simulink model "ResearchPaper4Fig9"  (R2015b)
settings: Solver=VariableStepAuto  StartTime=0.0  StopTime=10.0  RelTol=1e-3
libraries: xbsIndex_r4 x942, commfilt2 x1, commrandsrc3 x1, commdigbbndam3 x1
(part 6 of 6)

== system ResearchPaper4Fig9/PseudoConv. RVTDNN6/Output Neuron1/Weight Update4 for O.N ==
  eta'grad : Inport
  o1 : Inport  Port=2
  AddSub : xbsIndex_r4/AddSub  mode=Addition  use_carryin=off  use_carryout=off  en=off  latency=0  precision=Full  arith_type=Unsigned  n_bits=16  bin_pt=14  quantization=Truncate  overflow=Wrap  use_behavioral_HDL=off  hw_selection=Fabric  pipelined=off  dbl_ovrd=off  block_type=addsub
  Mult : xbsIndex_r4/Mult  precision=Full  arith_type="Signed  (2's comp)"  n_bits=16  bin_pt=14  quantization=Truncate  overflow=Wrap  en=off  latency=0  use_behavioral_HDL=off  opt=Speed  use_embedded=on  optimum_pipeline=off  pipeline=on  dbl_ovrd=off  use_rpm=on  placement_style=Triangular  block_type=mult
  Register : xbsIndex_r4/Register  init=0  rst=off  en=off  dbl_ovrd=off  block_type=register
  w11 : Outport
  wires:
  Mult/1 -> AddSub/1
  Register/1 -> w11/1, AddSub/2
  AddSub/1 -> Register/1
  eta'grad/1 -> Mult/1
  o1/1 -> Mult/2

== system ResearchPaper4Fig9/PseudoConv. RVTDNN6/Output Neuron1/Weight Update5 for O.N ==
  eta'grad : Inport
  o1 : Inport  Port=2
  AddSub : xbsIndex_r4/AddSub  mode=Addition  use_carryin=off  use_carryout=off  en=off  latency=0  precision=Full  arith_type=Unsigned  n_bits=16  bin_pt=14  quantization=Truncate  overflow=Wrap  use_behavioral_HDL=off  hw_selection=Fabric  pipelined=off  dbl_ovrd=off  block_type=addsub
  Mult : xbsIndex_r4/Mult  precision=Full  arith_type="Signed  (2's comp)"  n_bits=16  bin_pt=14  quantization=Truncate  overflow=Wrap  en=off  latency=0  use_behavioral_HDL=off  opt=Speed  use_embedded=on  optimum_pipeline=off  pipeline=on  dbl_ovrd=off  use_rpm=on  placement_style=Triangular  block_type=mult
  Register : xbsIndex_r4/Register  init=0  rst=off  en=off  dbl_ovrd=off  block_type=register
  w11 : Outport
  wires:
  Mult/1 -> AddSub/1
  Register/1 -> w11/1, AddSub/2
  AddSub/1 -> Register/1
  eta'grad/1 -> Mult/1
  o1/1 -> Mult/2

== system ResearchPaper4Fig9/PseudoConv. RVTDNN6/Output Neuron1/Weight Update6 for O.N ==
  eta'grad : Inport
  o1 : Inport  Port=2
  AddSub : xbsIndex_r4/AddSub  mode=Addition  use_carryin=off  use_carryout=off  en=off  latency=0  precision=Full  arith_type=Unsigned  n_bits=16  bin_pt=14  quantization=Truncate  overflow=Wrap  use_behavioral_HDL=off  hw_selection=Fabric  pipelined=off  dbl_ovrd=off  block_type=addsub
  Mult : xbsIndex_r4/Mult  precision=Full  arith_type="Signed  (2's comp)"  n_bits=16  bin_pt=14  quantization=Truncate  overflow=Wrap  en=off  latency=0  use_behavioral_HDL=off  opt=Speed  use_embedded=on  optimum_pipeline=off  pipeline=on  dbl_ovrd=off  use_rpm=on  placement_style=Triangular  block_type=mult
  Register : xbsIndex_r4/Register  init=0  rst=off  en=off  dbl_ovrd=off  block_type=register
  w11 : Outport
  wires:
  Mult/1 -> AddSub/1
  Register/1 -> w11/1, AddSub/2
  AddSub/1 -> Register/1
  eta'grad/1 -> Mult/1
  o1/1 -> Mult/2

== system ResearchPaper4Fig9/PseudoConv. RVTDNN6/Output Neuron2/Bias Update for O.N ==
  grad : Inport
  AddSub : xbsIndex_r4/AddSub  mode=Addition  use_carryin=off  use_carryout=off  en=off  latency=0  precision=Full  arith_type=Unsigned  n_bits=16  bin_pt=14  quantization=Truncate  overflow=Wrap  use_behavioral_HDL=off  hw_selection=Fabric  pipelined=off  dbl_ovrd=off  block_type=addsub
  Register : xbsIndex_r4/Register  init=0  rst=off  en=off  dbl_ovrd=off  block_type=register
  w10 : Outport
  wires:
  Register/1 -> w10/1, AddSub/2
  AddSub/1 -> Register/1
  grad/1 -> AddSub/1

== system ResearchPaper4Fig9/PseudoConv. RVTDNN6/Output Neuron2/Sum ==
  In1 : Inport
  In2 : Inport  Port=2
  In3 : Inport  Port=3
  In4 : Inport  Port=4
  In5 : Inport  Port=5
  In6 : Inport  Port=6
  In7 : Inport  Port=7
  AddSub{,1..5} (6 alike) : xbsIndex_r4/AddSub  mode=Addition  use_carryin=off  use_carryout=off  en=off  latency=0  precision=Full  arith_type=Unsigned  n_bits=16  bin_pt=14  quantization=Truncate  overflow=Wrap  use_behavioral_HDL=off  hw_selection=Fabric  pipelined=off  dbl_ovrd=off  block_type=addsub
  Out : Outport
  wires:
  AddSub4/1 -> AddSub5/2
  AddSub3/1 -> AddSub5/1
  In7/1 -> AddSub4/2
  AddSub1/1 -> AddSub3/2
  AddSub2/1 -> AddSub4/1
  In1/1 -> AddSub/1
  In6/1 -> AddSub2/2
  In2/1 -> AddSub/2
  In4/1 -> AddSub1/2
  AddSub/1 -> AddSub3/1
  In5/1 -> AddSub2/1
  AddSub5/1 -> Out/1
  In3/1 -> AddSub1/1

== system ResearchPaper4Fig9/PseudoConv. RVTDNN6/Output Neuron2/Weight Update1 for O.N ==
  eta'grad : Inport
  o1 : Inport  Port=2
  AddSub : xbsIndex_r4/AddSub  mode=Addition  use_carryin=off  use_carryout=off  en=off  latency=0  precision=Full  arith_type=Unsigned  n_bits=16  bin_pt=14  quantization=Truncate  overflow=Wrap  use_behavioral_HDL=off  hw_selection=Fabric  pipelined=off  dbl_ovrd=off  block_type=addsub
  Mult : xbsIndex_r4/Mult  precision=Full  arith_type="Signed  (2's comp)"  n_bits=16  bin_pt=14  quantization=Truncate  overflow=Wrap  en=off  latency=0  use_behavioral_HDL=off  opt=Speed  use_embedded=on  optimum_pipeline=off  pipeline=on  dbl_ovrd=off  use_rpm=on  placement_style=Triangular  block_type=mult
  Register : xbsIndex_r4/Register  init=0  rst=off  en=off  dbl_ovrd=off  block_type=register
  w11 : Outport
  wires:
  Mult/1 -> AddSub/1
  Register/1 -> w11/1, AddSub/2
  AddSub/1 -> Register/1
  eta'grad/1 -> Mult/1
  o1/1 -> Mult/2

== system ResearchPaper4Fig9/PseudoConv. RVTDNN6/Output Neuron2/Weight Update2 for O.N ==
  eta'grad : Inport
  o1 : Inport  Port=2
  AddSub : xbsIndex_r4/AddSub  mode=Addition  use_carryin=off  use_carryout=off  en=off  latency=0  precision=Full  arith_type=Unsigned  n_bits=16  bin_pt=14  quantization=Truncate  overflow=Wrap  use_behavioral_HDL=off  hw_selection=Fabric  pipelined=off  dbl_ovrd=off  block_type=addsub
  Mult : xbsIndex_r4/Mult  precision=Full  arith_type="Signed  (2's comp)"  n_bits=16  bin_pt=14  quantization=Truncate  overflow=Wrap  en=off  latency=0  use_behavioral_HDL=off  opt=Speed  use_embedded=on  optimum_pipeline=off  pipeline=on  dbl_ovrd=off  use_rpm=on  placement_style=Triangular  block_type=mult
  Register : xbsIndex_r4/Register  init=0  rst=off  en=off  dbl_ovrd=off  block_type=register
  w11 : Outport
  wires:
  Mult/1 -> AddSub/1
  Register/1 -> w11/1, AddSub/2
  AddSub/1 -> Register/1
  eta'grad/1 -> Mult/1
  o1/1 -> Mult/2

== system ResearchPaper4Fig9/PseudoConv. RVTDNN6/Output Neuron2/Weight Update3 for O.N ==
  eta'grad : Inport
  o1 : Inport  Port=2
  AddSub : xbsIndex_r4/AddSub  mode=Addition  use_carryin=off  use_carryout=off  en=off  latency=0  precision=Full  arith_type=Unsigned  n_bits=16  bin_pt=14  quantization=Truncate  overflow=Wrap  use_behavioral_HDL=off  hw_selection=Fabric  pipelined=off  dbl_ovrd=off  block_type=addsub
  Mult : xbsIndex_r4/Mult  precision=Full  arith_type="Signed  (2's comp)"  n_bits=16  bin_pt=14  quantization=Truncate  overflow=Wrap  en=off  latency=0  use_behavioral_HDL=off  opt=Speed  use_embedded=on  optimum_pipeline=off  pipeline=on  dbl_ovrd=off  use_rpm=on  placement_style=Triangular  block_type=mult
  Register : xbsIndex_r4/Register  init=0  rst=off  en=off  dbl_ovrd=off  block_type=register
  w11 : Outport
  wires:
  Mult/1 -> AddSub/1
  Register/1 -> w11/1, AddSub/2
  AddSub/1 -> Register/1
  eta'grad/1 -> Mult/1
  o1/1 -> Mult/2

== system ResearchPaper4Fig9/PseudoConv. RVTDNN6/Output Neuron2/Weight Update4 for O.N ==
  eta'grad : Inport
  o1 : Inport  Port=2
  AddSub : xbsIndex_r4/AddSub  mode=Addition  use_carryin=off  use_carryout=off  en=off  latency=0  precision=Full  arith_type=Unsigned  n_bits=16  bin_pt=14  quantization=Truncate  overflow=Wrap  use_behavioral_HDL=off  hw_selection=Fabric  pipelined=off  dbl_ovrd=off  block_type=addsub
  Mult : xbsIndex_r4/Mult  precision=Full  arith_type="Signed  (2's comp)"  n_bits=16  bin_pt=14  quantization=Truncate  overflow=Wrap  en=off  latency=0  use_behavioral_HDL=off  opt=Speed  use_embedded=on  optimum_pipeline=off  pipeline=on  dbl_ovrd=off  use_rpm=on  placement_style=Triangular  block_type=mult
  Register : xbsIndex_r4/Register  init=0  rst=off  en=off  dbl_ovrd=off  block_type=register
  w11 : Outport
  wires:
  Mult/1 -> AddSub/1
  Register/1 -> w11/1, AddSub/2
  AddSub/1 -> Register/1
  eta'grad/1 -> Mult/1
  o1/1 -> Mult/2

== system ResearchPaper4Fig9/PseudoConv. RVTDNN6/Output Neuron2/Weight Update5 for O.N ==
  eta'grad : Inport
  o1 : Inport  Port=2
  AddSub : xbsIndex_r4/AddSub  mode=Addition  use_carryin=off  use_carryout=off  en=off  latency=0  precision=Full  arith_type=Unsigned  n_bits=16  bin_pt=14  quantization=Truncate  overflow=Wrap  use_behavioral_HDL=off  hw_selection=Fabric  pipelined=off  dbl_ovrd=off  block_type=addsub
  Mult : xbsIndex_r4/Mult  precision=Full  arith_type="Signed  (2's comp)"  n_bits=16  bin_pt=14  quantization=Truncate  overflow=Wrap  en=off  latency=0  use_behavioral_HDL=off  opt=Speed  use_embedded=on  optimum_pipeline=off  pipeline=on  dbl_ovrd=off  use_rpm=on  placement_style=Triangular  block_type=mult
  Register : xbsIndex_r4/Register  init=0  rst=off  en=off  dbl_ovrd=off  block_type=register
  w11 : Outport
  wires:
  Mult/1 -> AddSub/1
  Register/1 -> w11/1, AddSub/2
  AddSub/1 -> Register/1
  eta'grad/1 -> Mult/1
  o1/1 -> Mult/2

== system ResearchPaper4Fig9/PseudoConv. RVTDNN6/Output Neuron2/Weight Update6 for O.N ==
  eta'grad : Inport
  o1 : Inport  Port=2
  AddSub : xbsIndex_r4/AddSub  mode=Addition  use_carryin=off  use_carryout=off  en=off  latency=0  precision=Full  arith_type=Unsigned  n_bits=16  bin_pt=14  quantization=Truncate  overflow=Wrap  use_behavioral_HDL=off  hw_selection=Fabric  pipelined=off  dbl_ovrd=off  block_type=addsub
  Mult : xbsIndex_r4/Mult  precision=Full  arith_type="Signed  (2's comp)"  n_bits=16  bin_pt=14  quantization=Truncate  overflow=Wrap  en=off  latency=0  use_behavioral_HDL=off  opt=Speed  use_embedded=on  optimum_pipeline=off  pipeline=on  dbl_ovrd=off  use_rpm=on  placement_style=Triangular  block_type=mult
  Register : xbsIndex_r4/Register  init=0  rst=off  en=off  dbl_ovrd=off  block_type=register
  w11 : Outport
  wires:
  Mult/1 -> AddSub/1
  Register/1 -> w11/1, AddSub/2
  AddSub/1 -> Register/1
  eta'grad/1 -> Mult/1
  o1/1 -> Mult/2
